simulink model "Model_Mk1"  (R2021b)
settings: Solver=VariableStepAuto  StartTime=0.0  StopTime=20  RelTol=1e-3
model workspace (MAT data in the model file):
  ICs = [0 0 0 0 0 0 0 0 0 0 0 0]
  MoI_Rocket = [2000  0  0; 0  2000  0; 0  0  2000]
  com = 25
  mass = 1
libraries: vrlib x4, sharedutil x2, aerolibutil x2, sharedtransform x1
settings Model: Creator=davis  LastModifiedBy=uncle

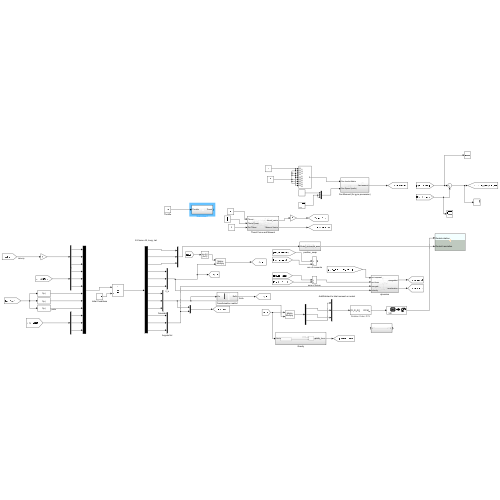
[thumbnail: Simulink's stored preview of the top-level diagram]
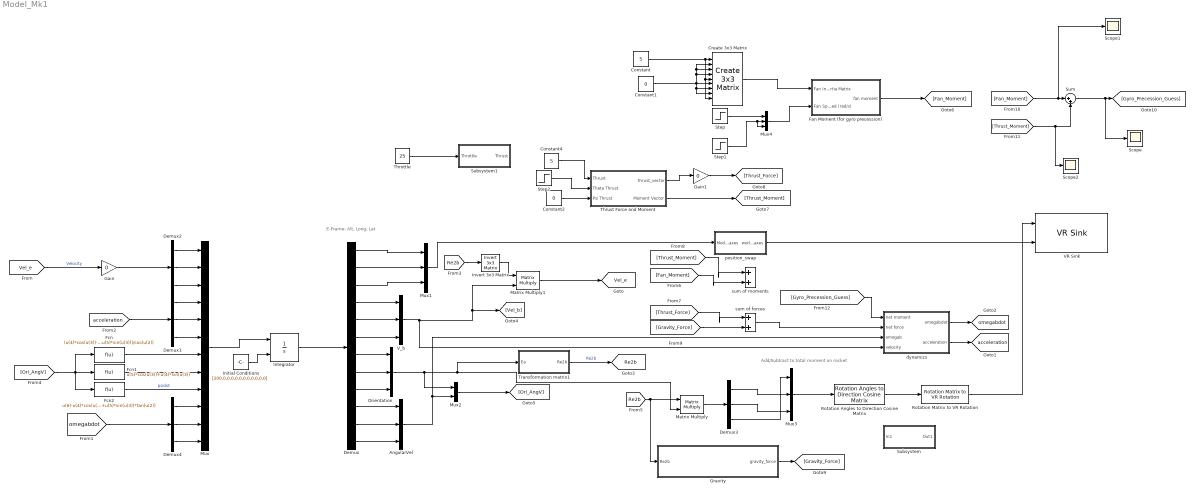
== system Model_Mk1 ==
  note: E-Frame: Alt, Long, Lat
  note: Add/Subtract to total moment on rocket
  AngularVel : Mux  Inputs=3
  Constant : Constant  Value=5
  Constant1 : Constant  Value=0
  Constant2 : Constant  Value=0
  Constant4 : Constant  Value=5
  Create 3x3 Matrix : sharedutil/Create 3x3 Matrix  aMode=aMode
      settings: SourceProductBaseCode=AE,PW,DR,MT,UV,VE
  Demux : Demux  Outputs=12
  Demux{1..4} (4 alike) : Demux  Outputs=3
  Fan Moment (for gyro precession) : Subsystem
  Fcn : Fcn  Expr=(u(4)*cos(u(3))-u(5)*sin(u(3)))/cos(u(2))
  Fcn1 : Fcn  Expr=u(5)*cos(u(3))+u(4)*sin(u(3))
  Fcn2 : Fcn  Expr=u(6)-u(4)*cos(u(3))*tan(u(2))+u(5)*sin(u(3))*tan(u(2))
  Gain : Gain  Gain=0
  Gain1 : Gain  Gain=0
  Gravity : Subsystem
  Initial Conditions : Constant  Value=[200,0,0,0,0,0,0,0,0,0,0,0]
  Integrator : Integrator  InitialConditionSource=external
  Invert 3x3 Matrix : aerolibutil/Invert  3x3 Matrix
  Matrix Multiply : Product  Multiplication=Matrix(*)
  Matrix Multiply1 : Product  Multiplication=Matrix(*)
  Mux : Mux  Inputs=12
  Mux1 : Mux  Inputs=3
  Mux2 : Mux  Inputs=2
  Mux3 : Mux  Inputs=3
  Mux4 : Mux  Inputs=3
  Orientation : Mux  Inputs=3
  Rotation Angles to Direction Cosine Matrix : sharedtransform/Rotation Angles to Direction Cosine Matrix  rotationOrder=ZYX  aMode=aMode
      settings: SourceProductBaseCode=AE,PW,DR,MT,UV,VE
  Rotation Matrix to VR Rotation : vrlib/Utilities/Rotation Matrix to VR Rotation  maxzero=1e-12
      settings: SourceProductBaseCode=SL
  Scope : Scope
  Scope1 : Scope
  Scope2 : Scope
  Step : Step  Time=5  Before=1  After=0  SampleTime=0
  Step1 : Step  Time=5  After=0  SampleTime=0
  Step2 : Step  Time=5  Before=pi/32  After=0  SampleTime=0
  Subsystem : Subsystem
  Subsystem1 : Subsystem
  Sum : Sum  Inputs=|++
  Throttle : Constant  Value=25
  Thrust Force and Moment : Subsystem
  Transformation matrix1 : Subsystem
  VR Sink : vrlib/VR Sink  InstantiateOnLoad=on  SampleTime=0.1  ViewEnable=on  RemoteChange=off  RemoteView=off  FieldsWritten=Rocket.rotation.4.1.1.double#Rocket.translation.3.1.1.double  WorldFileName=world.x3d  AutoView=off  VideoDimensions=[]  AllowVariableSize=off
  V_b : Mux  Inputs=3
  dynamics : Subsystem
  position_swap : Subsystem
  sum of forces : Sum  Inputs=|++
  sum of moments : Sum  Inputs=|++
  tag scope: Re2b=global, Vel_e=global, acceleration=global, omegabdot=global
  wires:
  Mux/1 -> Integrator/1
  Integrator/1 -> Demux/1
  Demux/1 -> Mux1/1
  Demux/2 -> Mux1/2
  Demux/3 -> Mux1/3
  Demux/4 -> V_b/1
  Demux/5 -> V_b/2
  Demux/6 -> V_b/3
  V_b/1 -> [Vel_b], Matrix Multiply1/2, dynamics/4(velocity)
  Demux1/1 -> Mux/4
  Demux1/2 -> Mux/5
  Demux1/3 -> Mux/6
  Demux2/1 -> Mux/1
  Demux2/3 -> Mux/3
  Demux2/2 -> Mux/2
  Initial Conditions/1 -> Integrator/2
  [acceleration] -> Demux1/1
  Fcn/1 -> Mux/7
  Fcn1/1 -> Mux/8
  Demux4/1 -> Mux/10
  Demux4/3 -> Mux/12
  [omegabdot] -> Demux4/1
  Demux4/2 -> Mux/11
  Demux/8 -> Orientation/2
  Demux/9 -> Orientation/3
  Demux/7 -> Orientation/1
  Demux/11 -> AngularVel/2
  AngularVel/1 -> Mux2/2, dynamics/3(omegab)
  Demux/12 -> AngularVel/3
  Demux/10 -> AngularVel/1
  dynamics/2(acceleration) -> [acceleration]
  dynamics/1(omegabdot) -> [omegabdot]
  Transformation matrix1/1(Re2b) -> [Re2b]  "Re2b"
  [Vel_e] -> Gain/1  "Velocity"
  Matrix Multiply1/1 -> [Vel_e]
  [Re2b] -> Invert 3x3 Matrix/1
  Invert 3x3 Matrix/1 -> Matrix Multiply1/1
  Fcn2/1 -> Mux/9  "psidot"
  Mux2/1 -> [Ori_AngV]
  [Ori_AngV] -> Fcn2/1, Fcn/1, Fcn1/1
  Demux3/1 -> Mux3/2
  Demux3/2 -> Mux3/3
  Demux3/3 -> Mux3/1
  [Re2b] -> Matrix Multiply/1, Gravity/1(Re2b)
  Matrix Multiply/1 -> Demux3/1
  Mux1/1 -> position_swap/1(Model_axes)
  Mux3/1 -> Rotation Angles to Direction Cosine Matrix/1
  Orientation/1 -> Transformation matrix1/1(Ea), Matrix Multiply/2, Mux2/1
  Rotation Angles to Direction Cosine Matrix/1 -> Rotation Matrix to VR Rotation/1
  Rotation Matrix to VR Rotation/1 -> VR Sink/1
  position_swap/1(world_axes) -> VR Sink/2
  Constant2/1 -> Thrust Force and Moment/3(Psi Thrust)
  Step2/1 -> Thrust Force and Moment/2(Theta Thrust)
  Constant4/1 -> Thrust Force and Moment/1(Thrust)
  sum of forces/1 -> dynamics/2(net force)
  [Fan_Moment] -> sum of moments/2
  [Thrust_Force] -> sum of forces/1
  [Thrust_Moment] -> sum of moments/1
  Gravity/1(gravity_force) -> [Gravity_Force]
  [Gravity_Force] -> sum of forces/2
  Step1/1 -> Mux4/3, Mux4/2
  Step/1 -> Mux4/1
  Constant1/1 -> Create 3x3 Matrix/6, Create 3x3 Matrix/7, Create 3x3 Matrix/8, Create 3x3 Matrix/4, Create 3x3 Matrix/3, Create 3x3 Matrix/2
  Constant/1 -> Create 3x3 Matrix/5, Create 3x3 Matrix/9, Create 3x3 Matrix/1
  Create 3x3 Matrix/1 -> Fan Moment (for gyro precession)/1(Fan Inertia Matrix)
  Mux4/1 -> Fan Moment (for gyro precession)/2(Fan Speed (rad/s))
  Gain/1 -> Demux2/1
  Thrust Force and Moment/1(thrust_vector) -> Gain1/1
  Gain1/1 -> [Thrust_Force]
  Thrust Force and Moment/2(Moment Vector) -> [Thrust_Moment]
  [Fan_Moment] -> Scope1/1, Sum/1
  [Thrust_Moment] -> Scope2/1, Sum/2
  Sum/1 -> Scope/1, [Gyro_Precession_Guess]
  [Gyro_Precession_Guess] -> dynamics/1(net moment)
  Fan Moment (for gyro precession)/1(fan moment) -> [Fan_Moment]
  Throttle/1 -> Subsystem1/1(Throttle)

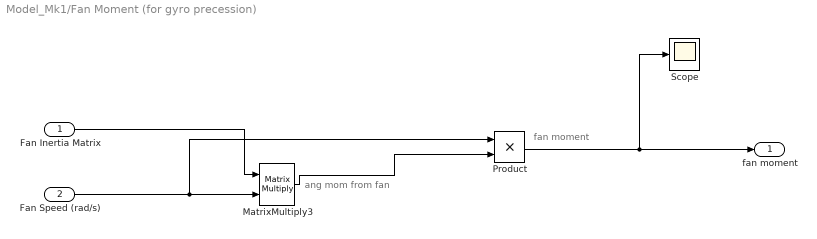
== system Model_Mk1/Fan Moment (for gyro precession) ==
  note: ang mom from fan
  note: fan moment
  Fan Inertia Matrix : Inport
  Fan Speed (rad/s) : Inport  Port=2
  MatrixMultiply3 : Product  Multiplication=Matrix(*)
  Product : Product
  Scope : Scope
  fan moment : Outport
  wires:
  Fan Inertia Matrix/1 -> MatrixMultiply3/1
  Product/1 -> Scope/1, fan moment/1
  Fan Speed (rad/s)/1 -> Product/1, MatrixMultiply3/2
  MatrixMultiply3/1 -> Product/2

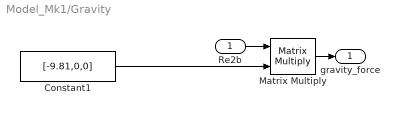
== system Model_Mk1/Gravity ==
  Re2b : Inport
  Constant1 : Constant  Value=[-9.81,0,0]
  Matrix Multiply : Product  Multiplication=Matrix(*)
  gravity_force : Outport
  wires:
  Matrix Multiply/1 -> gravity_force/1
  Re2b/1 -> Matrix Multiply/1
  Constant1/1 -> Matrix Multiply/2

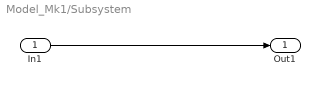
== system Model_Mk1/Subsystem ==
  In1 : Inport
  Out1 : Outport
  wires:
  In1/1 -> Out1/1

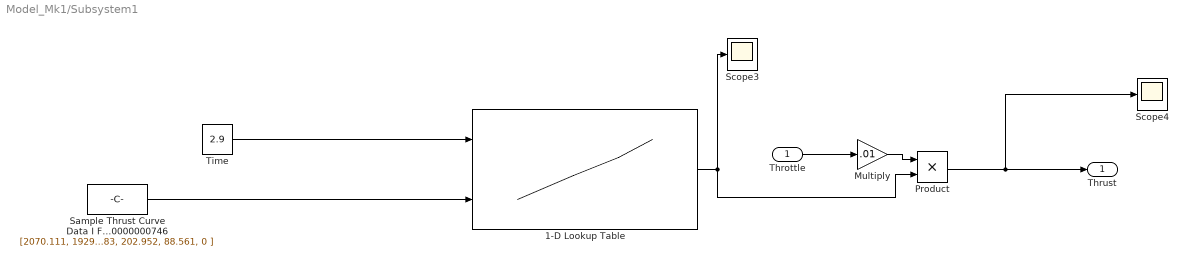
== system Model_Mk1/Subsystem1 ==
  Throttle : Inport
  1-D Lookup Table : Lookup_n-D  NumberOfTableDimensions=1  LookupTableObject=Lab 4.xlsx  BreakpointsForDimension1=[0:1:29]  TableSource=Input port  Table=[5,6,6.5,6.75,6.9,7]  InternalRulePriority=Speed  RndMeth=Simplest  InputSameDT=on
      settings: InputPortMap=u0,p221
  Multiply : Gain  Gain=.01
  Product : Product
  Sample Thrust Curve Data I Found Online https://www.thrustcurve.org/simfiles/5f4294d20002e90000000746 : Constant  Value=|
      | [2070.111,
      | 1929.889,
      | 2147.601,
      | 2369.004,
      | 2505.535,
      | 2649.446,
      | 2627.306,
      | 2608.856,
      | 2616.236,
      | 2623.616,
      | 2575.646,
      | 2538.745,
      | 2450.185,
      | 2394.834,
      | 2295.203,
      | 2206.642,
      | 2162.362,
      | 2088.561,
      | 1988.93,
      | 1800.738,
      | 1594.096,
      | 1335.793,
      | 1014.76,
      | 708.487,
      | 601.476,
      | 461.255,
      | 339.483,
      | 202.952,
      | 88.561,
      | 0
      | ]
  Scope3 : Scope
  Scope4 : Scope
  Time : Constant  Value=2.9
  Thrust : Outport
  wires:
  Sample Thrust Curve Data I Found Online https://www.thrustcurve.org/simfiles/5f4294d20002e90000000746/1 -> 1-D Lookup Table/2
  Time/1 -> 1-D Lookup Table/1
  Multiply/1 -> Product/1
  Throttle/1 -> Multiply/1
  Product/1 -> Scope4/1, Thrust/1
  1-D Lookup Table/1 -> Scope3/1, Product/2

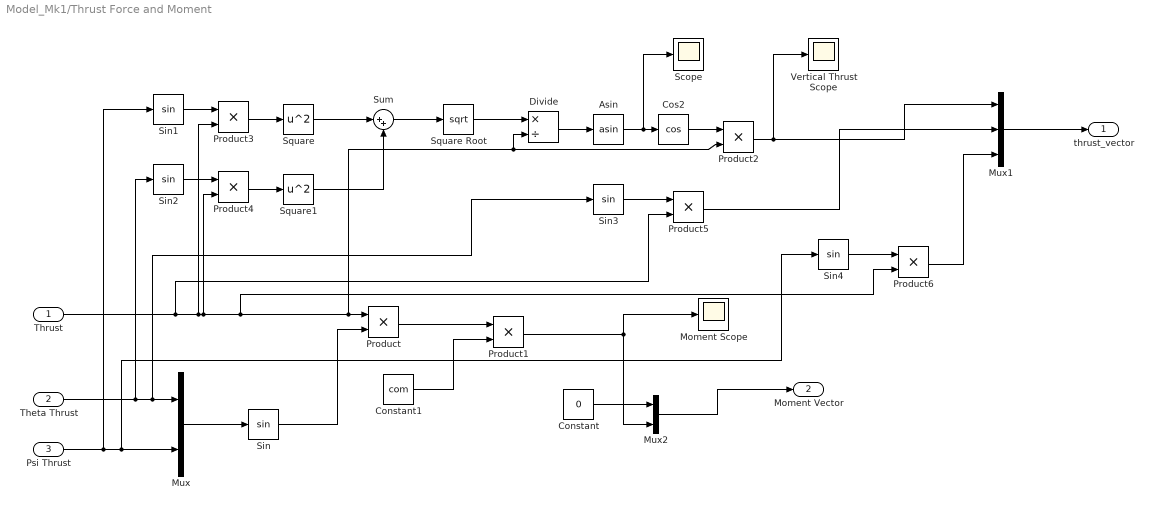
== system Model_Mk1/Thrust Force and Moment ==
  Thrust : Inport
  Theta Thrust : Inport  Port=2
  Psi Thrust : Inport  Port=3
  Asin : Trigonometry  Operator=asin
  Constant : Constant  Value=0
  Constant1 : Constant  Value=com
  Cos2 : Trigonometry  Operator=cos
  Divide : Product  Inputs=*/
  Moment Scope : Scope
  Mux : Mux  Inputs=2
  Mux1 : Mux  Inputs=3
  Mux2 : Mux  Inputs=2
  Product{,1..6} (7 alike) : Product
  Scope : Scope
  Sin{,1..4} (5 alike) : Trigonometry
  Square : Math  Operator=square  SaturateOnIntegerOverflow=on
  Square Root : Sqrt  SaturateOnIntegerOverflow=on
  Square1 : Math  Operator=square  SaturateOnIntegerOverflow=on
  Sum : Sum  Inputs=|++
  Vertical Thrust Scope : Scope
  thrust_vector : Outport
  Moment Vector : Outport  Port=2
  wires:
  Product2/1 -> Vertical Thrust Scope/1, Mux1/1
  Product1/1 -> Moment Scope/1, Mux2/2
  Product/1 -> Product1/1
  Constant1/1 -> Product1/2
  Sin/1 -> Product/2
  Asin/1 -> Cos2/1, Scope/1
  Cos2/1 -> Product2/1
  Divide/1 -> Asin/1
  Mux/1 -> Sin/1
  Product3/1 -> Square/1
  Product4/1 -> Square1/1
  Psi Thrust/1 -> Sin4/1, Mux/2, Sin1/1
  Sin1/1 -> Product3/1
  Sin2/1 -> Product4/1
  Square1/1 -> Sum/2
  Square/1 -> Sum/1
  Sum/1 -> Square Root/1
  Theta Thrust/1 -> Sin3/1, Mux/1, Sin2/1
  Thrust/1 -> Product5/2, Product6/2, Product2/2, Divide/2, Product/1, Product4/2, Product3/2
  Square Root/1 -> Divide/1
  Mux1/1 -> thrust_vector/1
  Sin3/1 -> Product5/1
  Product5/1 -> Mux1/2
  Sin4/1 -> Product6/1
  Product6/1 -> Mux1/3
  Mux2/1 -> Moment Vector/1
  Constant/1 -> Mux2/1

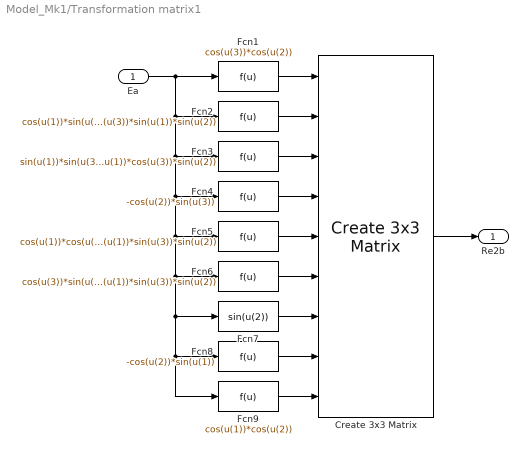
== system Model_Mk1/Transformation matrix1 ==
  Ea : Inport
  Create 3x3 Matrix : sharedutil/Create 3x3 Matrix  aMode=aMode
      settings: SourceProductBaseCode=AE,PW,DR,MT,UV,VE
  Fcn1 : Fcn  Expr=cos(u(3))*cos(u(2))
  Fcn2 : Fcn  Expr=cos(u(1))*sin(u(3)) + cos(u(3))*sin(u(1))*sin(u(2))
  Fcn3 : Fcn  Expr=sin(u(1))*sin(u(3)) - cos(u(1))*cos(u(3))*sin(u(2))
  Fcn4 : Fcn  Expr=-cos(u(2))*sin(u(3))
  Fcn5 : Fcn  Expr=cos(u(1))*cos(u(3)) - sin(u(1))*sin(u(3))*sin(u(2))
  Fcn6 : Fcn  Expr=cos(u(3))*sin(u(1)) + cos(u(1))*sin(u(3))*sin(u(2))
  Fcn7 : Fcn  Expr=sin(u(2))
  Fcn8 : Fcn  Expr=-cos(u(2))*sin(u(1))
  Fcn9 : Fcn  Expr=cos(u(1))*cos(u(2))
  Re2b : Outport  VectorParamsAs1DForOutWhenUnconnected=off
  wires:
  Ea/1 -> Fcn9/1, Fcn8/1, Fcn7/1, Fcn6/1, Fcn5/1, Fcn4/1, Fcn3/1, Fcn2/1, Fcn1/1
  Fcn9/1 -> Create 3x3 Matrix/9
  Fcn8/1 -> Create 3x3 Matrix/8
  Fcn7/1 -> Create 3x3 Matrix/7
  Fcn6/1 -> Create 3x3 Matrix/6
  Fcn5/1 -> Create 3x3 Matrix/5
  Fcn4/1 -> Create 3x3 Matrix/4
  Fcn3/1 -> Create 3x3 Matrix/3
  Fcn2/1 -> Create 3x3 Matrix/2
  Fcn1/1 -> Create 3x3 Matrix/1
  Create 3x3 Matrix/1 -> Re2b/1

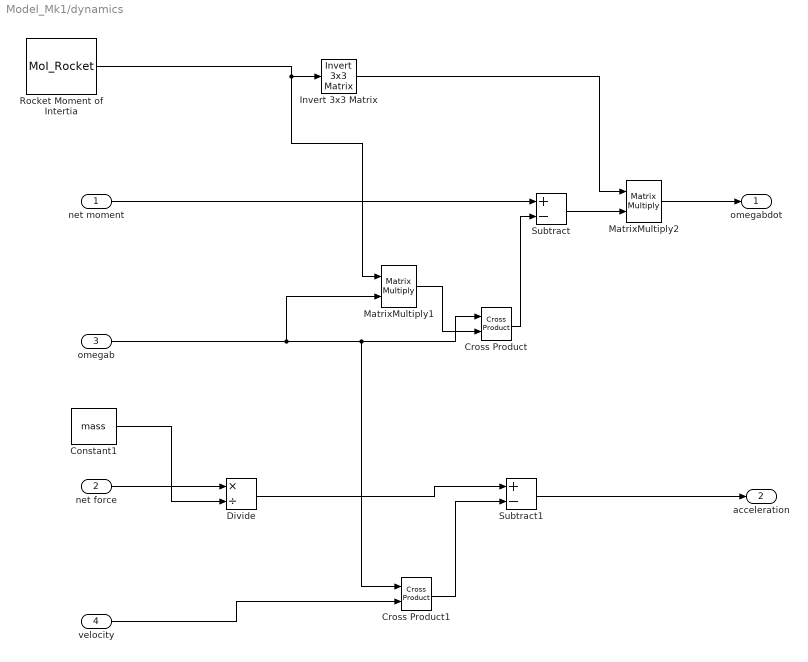
== system Model_Mk1/dynamics ==
  net moment : Inport
  net force : Inport  Port=2
  omegab : Inport  Port=3
  velocity : Inport  Port=4
  Constant1 : Constant  Value=mass
  Cross Product : vrlib/Utilities/Cross Product
  Cross Product1 : vrlib/Utilities/Cross Product
  Divide : Product  Inputs=*/
  Invert 3x3 Matrix : aerolibutil/Invert  3x3 Matrix
  MatrixMultiply1 : Product  Multiplication=Matrix(*)
  MatrixMultiply2 : Product  Multiplication=Matrix(*)
  Rocket Moment of Intertia : Constant  Value=MoI_Rocket
  Subtract : Sum  Inputs=+-
  Subtract1 : Sum  Inputs=+-
  omegabdot : Outport
  acceleration : Outport  Port=2
  wires:
  Rocket Moment of Intertia/1 -> MatrixMultiply1/1, Invert 3x3 Matrix/1
  net moment/1 -> Subtract/1
  omegab/1 -> Cross Product1/1, Cross Product/1, MatrixMultiply1/2
  Cross Product/1 -> Subtract/2
  Subtract/1 -> MatrixMultiply2/2
  Invert 3x3 Matrix/1 -> MatrixMultiply2/1
  MatrixMultiply2/1 -> omegabdot/1
  MatrixMultiply1/1 -> Cross Product/2
  Constant1/1 -> Divide/2
  net force/1 -> Divide/1
  Divide/1 -> Subtract1/1
  velocity/1 -> Cross Product1/2
  Cross Product1/1 -> Subtract1/2
  Subtract1/1 -> acceleration/1

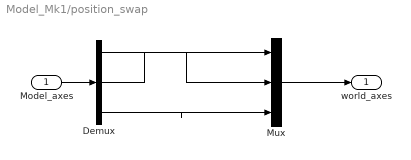
== system Model_Mk1/position_swap ==
  Model_axes : Inport
  Demux : Demux  Outputs=3
  Mux : Mux  Inputs=3
  world_axes : Outport
  wires:
  Demux/3 -> Mux/3
  Demux/2 -> Mux/1
  Mux/1 -> world_axes/1
  Demux/1 -> Mux/2
  Model_axes/1 -> Demux/1
